simulink model "nodes2"  (R2014a)
settings: Solver=ode45  SolverMode=SingleTasking  StartTime=0.0  StopTime=tstop  FixedStep=ts  RelTol=1e-3
values from neighbouring files (symbols this model uses):
  data_rate = 0.1    [llencadora_sim.m]
  num_generators = tot    (= 8)    [llencadora_sim.m]
  num_loads = tot    (= 8)    [llencadora_sim.m]
  ts = 100e-6    (= 0.0001)    [llencadora_sim.m]    (also in processor.m = data.ts)
libraries: experiment_lib2 x5, truetime x1, experiment_lib x1, powerlib x1
settings Model: SimulationMode=accelerator  ExtModeTrigDuration=100  Creator=sepic  LastModifiedBy=mvelasco
settings SolverCC: MaxConsecutiveMinStep=1000
settings DataIOCC: SaveFinalState=on  SaveFormat=StructureWithTime  SignalLoggingSaveFormat=ModelDataLogs  SaveOutput=off  SaveState=on  StateSaveName=tmp_raccel_xout  SignalLoggingName=tmp_raccel_logsout
settings OptimizationCC: ExpressionDepthLimit=2147483647  InitFltsAndDblsToZero=on  EfficientMapNaN2IntZero=off
settings DebuggingCC: ReadBeforeWriteMsg=DisableAll  WriteAfterWriteMsg=DisableAll  WriteAfterReadMsg=DisableAll  UnderspecifiedInitializationDetection=Classic  MultiTaskDSMMsg=none  FcnCallInpInsideContextMsg=UseLocalSettings  StateNameClashWarn=warning
settings HardwareCC: TargetBitPerLong=64  TargetBitPerPointer=64  TargetLongLongMode=on  TargetIntDivRoundTo=Zero  TargetEndianess=LittleEndian  TargetWordSize=64  TargetHWDeviceType=MATLAB Host  ProdEqTarget=off
settings SFSimCC: SimParseCustomCode=off
settings RTWCC: SystemTargetFile=raccel.tlc  TemplateMakefile=raccel_default_tmf  RTWVerbose=off  ProcessScript=raccel_make_rtw_hook  RTWUseSimCustomCode=on  TargetLang=C++
settings CodeAppCC: GenerateComments=off  MaxIdLength=128  MangleLength=10  SimulinkBlockComments=off
settings RaccelTargetCC: ERTMultiwordTypeDef=System defined  ERTMultiwordLength=256  GeneratePreprocessorConditionals=Disable all  ERTFirstTimeCompliant=off  MultiInstanceERTCode=off  EnableShiftOperators=on  ENABLE_SLEXEC_SSBRIDGE=0  RTWCAPIParams=off

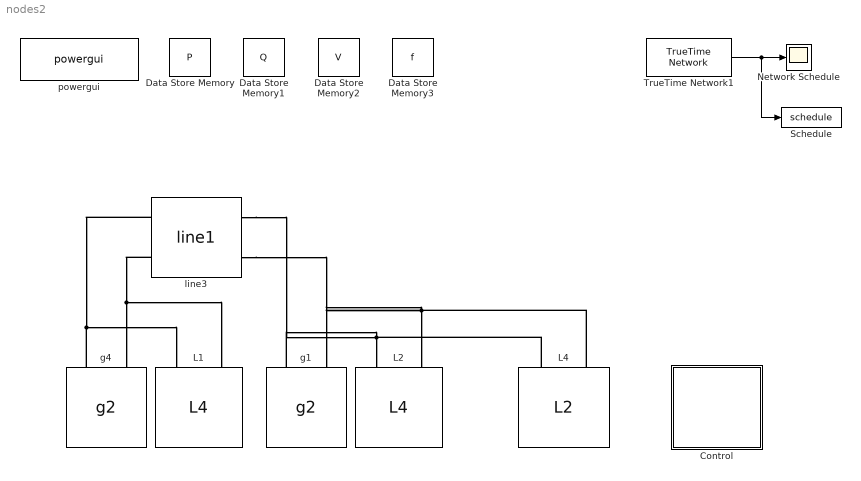
== system nodes2 ==
  Control : Subsystem
  Data Store Memory : DataStoreMemory  DataStoreName=P  ReadBeforeWriteMsg=warning  WriteAfterWriteMsg=warning  WriteAfterReadMsg=warning  InitialValue=zeros(1,num_generators)
  Data Store Memory1 : DataStoreMemory  DataStoreName=Q  ReadBeforeWriteMsg=warning  WriteAfterWriteMsg=warning  WriteAfterReadMsg=warning  InitialValue=zeros(1,num_generators)
  Data Store Memory2 : DataStoreMemory  DataStoreName=V  ReadBeforeWriteMsg=warning  WriteAfterWriteMsg=warning  WriteAfterReadMsg=warning  InitialValue=zeros(1,num_generators)
  Data Store Memory3 : DataStoreMemory  DataStoreName=f  ReadBeforeWriteMsg=warning  WriteAfterWriteMsg=warning  WriteAfterReadMsg=warning  InitialValue=zeros(1,num_generators)
  L1 : experiment_lib2/L4  a=1
  L2 : experiment_lib2/L4  a=2
  L4 : experiment_lib2/L2  a=1
  Network Schedule : Scope
      settings: TimeRange=2  YMin=1  YMax=2.5  SaveName=nschedule1
  Schedule : ToWorkspace  VariableName=schedule  SaveFormat=Structure With Time  SampleTime=-1
  TrueTime Network1 : truetime/TrueTime Network  nwtype=CSMA/CD (Ethernet)  nwnbr=1  nnodes=num_generators+1  rate=100e6  minsize=80  lossprob=loss  seed=0  bandwidths=[0.5 0.25 0.25]  slotsize=80  schedule=[1 2 1 3]  memsize=80000  buftype=Common buffer  overflow=Retransmit  dynSchedule=0  miniSlotSize=0  NIT=0  QSortMode=FIFO  sync=0  irtSchedule=0  nrtLength=0  nodeGraph=0  scheduleoutput=on
  g1 : experiment_lib2/g2  a=2
  g4 : experiment_lib2/g2  a=1
  line3 : experiment_lib/line1  a=1
  powergui : powerlib/powergui  SimulationMode=Continuous  SolverType=Tustin  SampleTime=ts  frequency=60  SPID=off  DisableSnubberDevices=off  DisableRonSwitches=off  DisableVfSwitches=off  SwTol=0  Interpol=off  DisplayEquations=off  Ts=0  methode=off  frequencyindice=0  Pbase=100e6  ErrMax=1e-4  Iterations=50  UnitsV=kV  UnitsW=MW  FunctionMessages=off  echomessages=off  HookPort=off  EnableUseOfTLC=off  x0status=blocks  RestoreLinks=warning  ResistiveCurrentMeasurement=off  Frange=[0:2:500]  Ylog=off  Xlog=on  ShowGrid=off  save=off  variable=ZData  structure=0  ZoomFFT=on  StartTime=0.0  cycles=1  DisplayStyle=1  fundamental=60  FreqAxis=off  MaxFrequency=1000  frequencyindicesteady=1  RmsSteady=1  display=off
  wires:
  TrueTime Network1/1 -> Network Schedule/1, Schedule/1
  connections:
  line3/LConn1 -- g1/LConn1 -- L4/LConn1 -- L2/LConn1
  line3/LConn2 -- g1/LConn2 -- L4/LConn2 -- L2/LConn2
  line3/RConn1 -- g4/LConn1 -- L1/LConn1
  line3/RConn2 -- g4/LConn2 -- L1/LConn2

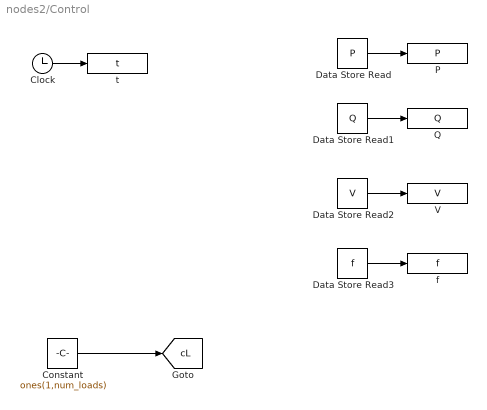
== system nodes2/Control ==
  Clock : Clock
  Constant : Constant  Value=ones(1,num_loads)
  Data Store Read : DataStoreRead  DataStoreName=P  SampleTime=0
  Data Store Read1 : DataStoreRead  DataStoreName=Q  SampleTime=0
  Data Store Read2 : DataStoreRead  DataStoreName=V  SampleTime=0
  Data Store Read3 : DataStoreRead  DataStoreName=f  SampleTime=0
  P : ToWorkspace  VariableName=P  SampleTime=data_rate
  Q : ToWorkspace  VariableName=Q  SampleTime=data_rate
  V : ToWorkspace  VariableName=V  SampleTime=data_rate
  f : ToWorkspace  VariableName=f  SampleTime=data_rate
  t : ToWorkspace  VariableName=t  SampleTime=data_rate
  tag scope: cL=global
  wires:
  Clock/1 -> t/1
  Data Store Read/1 -> P/1
  Data Store Read1/1 -> Q/1
  Data Store Read2/1 -> V/1
  Data Store Read3/1 -> f/1
  Constant/1 -> [cL]
